simulink model "Pacemaker_Deliverable_1_Final_2023a"  (R2023a)
settings: Solver=FixedStepAuto  StartTime=0.0  StopTime=10.0  FixedStep=1e-3  RelTol=1e-3  EnableMultiTasking=on
undefined symbols (not defined in the file): D0, D1, D10, D11, D12, D13, D2, D3, D5, D6, D8, D9, PTA0, PTA1, PTA2, PTB9, PTC16, PTC17, PTC2, PTC4, PTD0, PTD1, PTD2, PTD3
libraries: frdmk64flib x14
settings Model: ExtModeTrigDuration=5  Creator=kelby  LastModifiedBy=kelby
settings OptimizationCC: EnhancedBackFolding=on  PassReuseOutputArgsAs=Individual arguments  ZeroExternalMemoryAtStartup=off  ZeroInternalMemoryAtStartup=off  MaxStackSize=64  OptimizeBlockOrder=speed  DifferentSizesBufferReuse=on  OptimizationCustomize=off  EfficientTunableParamExpr=on
settings DebuggingCC: ParameterTunabilityLossMsg=error
settings HardwareCC: ProdBitPerPointer=32  ProdBitPerSizeT=32  ProdBitPerPtrDiffT=32  ProdLargestAtomicInteger=Long  ProdLargestAtomicFloat=Double  ProdWordSize=32  ProdHWDeviceType=ARM Compatible->ARM Cortex
settings SFSimCC: MATLABDynamicMemAlloc=off
settings RTWCC: Description=Embedded Coder  SystemTargetFile=ert.tlc  HardwareBoard=NXP FRDM-K64F  TLCOptions="-aInlineSetEventsForThisBaseRateFcn=TLC_FALSE -aSuppressMultiTaskScheduler=TLC_FALSE  -aRateBasedStepFcn=0"  TemplateMakefile=ert_default_tmf  Toolchain=GNU Tools for ARM Embedded Processors
settings CodeAppCC: ForceParamTrailComments=on  IgnoreCustomStorageClasses=off  OperatorAnnotations=on  SimulinkDataObjDesc=on  SFDataObjDesc=on  InsertBlockDesc=on
settings ERTTargetCC: ExtModeTransport=4  ExtModeMexFile=sendToCommService

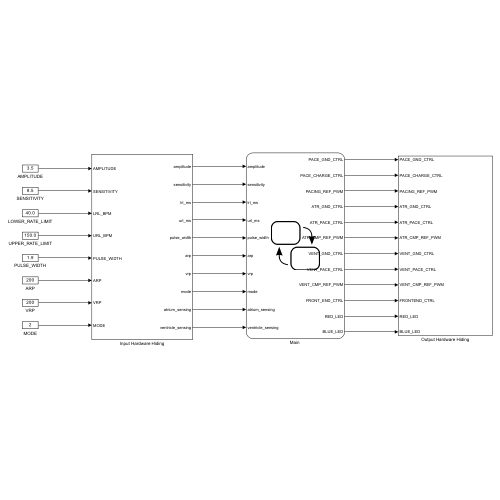
[thumbnail: Simulink's stored preview of the top-level diagram]
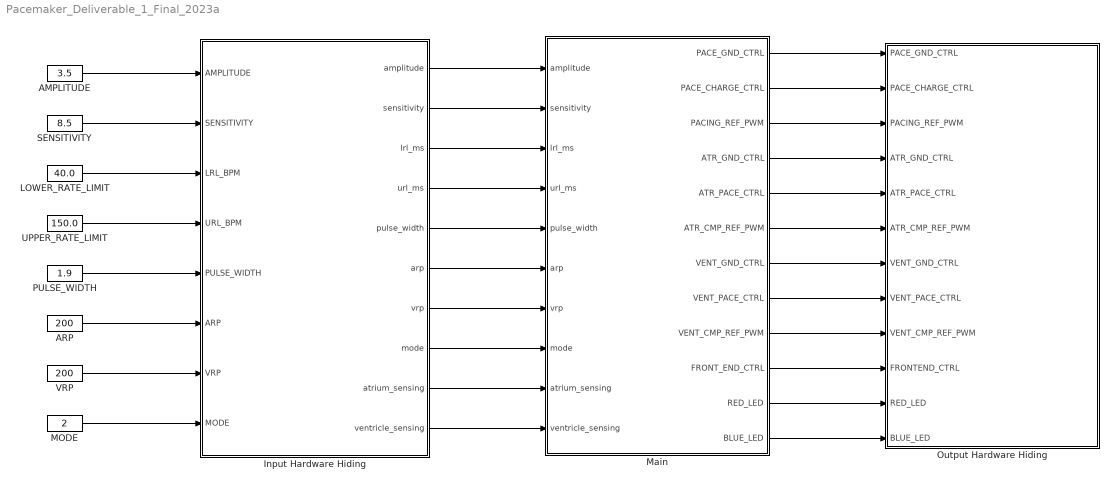
== system Pacemaker_Deliverable_1_Final_2023a ==
  AMPLITUDE : Constant  Value=3.5
  ARP : Constant  Value=200
  Input Hardware Hiding : Subsystem
  LOWER_RATE_LIMIT : Constant  Value=40.0
  MODE : Constant  Value=2
  "Main " : Stateflow chart  TreatAsAtomicUnit=on
  Output Hardware Hiding : Subsystem
  PULSE_WIDTH : Constant  Value=1.9
  SENSITIVITY : Constant  Value=8.5
  UPPER_RATE_LIMIT : Constant  Value=150.0
  VRP : Constant  Value=200
  wires:
  Input Hardware Hiding/1(amplitude) -> "Main "/1(amplitude)
  Input Hardware Hiding/3(lrl_ms) -> "Main "/3(lrl_ms)
  Input Hardware Hiding/4(url_ms) -> "Main "/4(url_ms)
  Input Hardware Hiding/5(pulse_width) -> "Main "/5(pulse_width)
  Input Hardware Hiding/8(mode) -> "Main "/8(mode)
  Input Hardware Hiding/6(arp) -> "Main "/6(arp)
  Input Hardware Hiding/7(vrp) -> "Main "/7(vrp)
  Input Hardware Hiding/2(sensitivity) -> "Main "/2(sensitivity)
  "Main "/4(ATR_GND_CTRL) -> Output Hardware Hiding/4(ATR_GND_CTRL)
  "Main "/5(ATR_PACE_CTRL) -> Output Hardware Hiding/5(ATR_PACE_CTRL)
  "Main "/2(PACE_CHARGE_CTRL) -> Output Hardware Hiding/2(PACE_CHARGE_CTRL)
  "Main "/1(PACE_GND_CTRL) -> Output Hardware Hiding/1(PACE_GND_CTRL)
  "Main "/3(PACING_REF_PWM) -> Output Hardware Hiding/3(PACING_REF_PWM)
  "Main "/7(VENT_GND_CTRL) -> Output Hardware Hiding/7(VENT_GND_CTRL)
  "Main "/8(VENT_PACE_CTRL) -> Output Hardware Hiding/8(VENT_PACE_CTRL)
  "Main "/9(VENT_CMP_REF_PWM) -> Output Hardware Hiding/9(VENT_CMP_REF_PWM)
  "Main "/6(ATR_CMP_REF_PWM) -> Output Hardware Hiding/6(ATR_CMP_REF_PWM)
  "Main "/12(BLUE_LED) -> Output Hardware Hiding/12(BLUE_LED)
  "Main "/11(RED_LED) -> Output Hardware Hiding/11(RED_LED)
  AMPLITUDE/1 -> Input Hardware Hiding/1(AMPLITUDE)
  LOWER_RATE_LIMIT/1 -> Input Hardware Hiding/3(LRL_BPM)
  UPPER_RATE_LIMIT/1 -> Input Hardware Hiding/4(URL_BPM)
  PULSE_WIDTH/1 -> Input Hardware Hiding/5(PULSE_WIDTH)
  MODE/1 -> Input Hardware Hiding/8(MODE)
  ARP/1 -> Input Hardware Hiding/6(ARP)
  VRP/1 -> Input Hardware Hiding/7(VRP)
  SENSITIVITY/1 -> Input Hardware Hiding/2(SENSITIVITY)
  Input Hardware Hiding/9(atrium_sensing) -> "Main "/9(atrium_sensing)
  Input Hardware Hiding/10(ventricle_sensing) -> "Main "/10(ventricle_sensing)
  "Main "/10(FRONT_END_CTRL) -> Output Hardware Hiding/10(FRONTEND_CTRL)

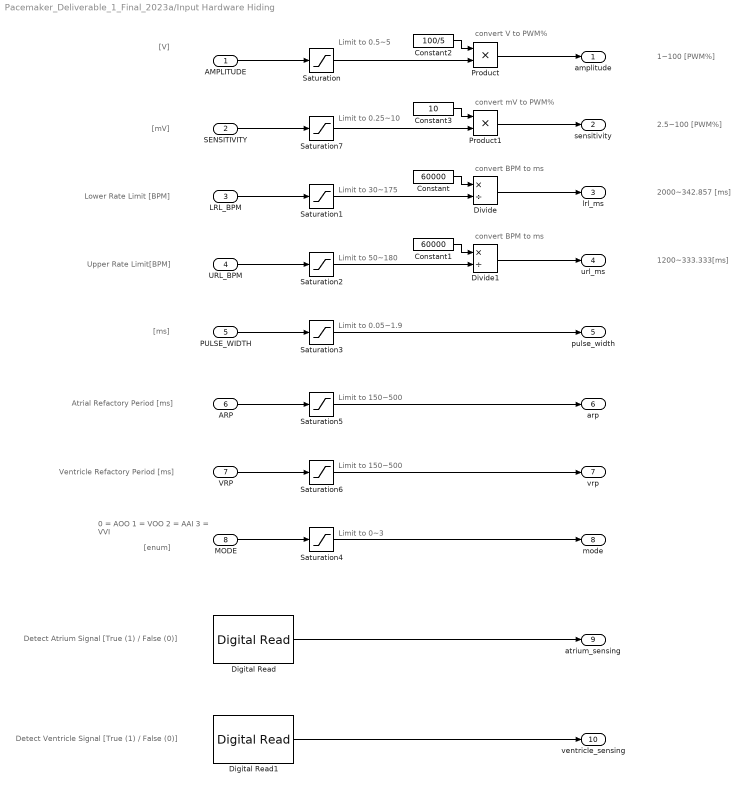
== system Pacemaker_Deliverable_1_Final_2023a/Input Hardware Hiding ==
  note: 0 = AOO
      | 1 = VOO
      | 2 = AAI
      | 3 = VVI
  note: Detect Atrium Signal [True (1) / False (0)]
  note: Limit to 0.5~5
  note: convert BPM to ms
  note: Ventricle Refactory Period [ms]
  note: Atrial Refactory Period [ms]
  note: convert BPM to ms
  note: Limit to 30~175
  note: Limit to 50~180
  note: Limit to 0.05~1.9
  note: Limit to 0~3
  note: Limit to 150~500
  note: Limit to 150~500
  note: Limit to 0.25~10
  note: convert V to PWM%
  note: convert mV to PWM%
  note: [mV]
  note: 2.5~100 [PWM%]
  note: 1~100 [PWM%]
  note: Lower Rate Limit [BPM]
  note: Upper Rate Limit[BPM]
  note: 2000~342.857 [ms]
  note: 1200~333.333[ms]
  note: [ms]
  note: [enum]
  note: [V]
  note: Detect Ventricle Signal [True (1) / False (0)]
  AMPLITUDE : Inport
  SENSITIVITY : Inport  Port=2
  LRL_BPM : Inport  Port=3
  URL_BPM : Inport  Port=4
  PULSE_WIDTH : Inport  Port=5
  ARP : Inport  Port=6
  VRP : Inport  Port=7
  MODE : Inport  Port=8
  Constant : Constant  Value=60000
  Constant1 : Constant  Value=60000
  Constant2 : Constant  Value=100/5
  Constant3 : Constant  Value=10
  Digital Read : frdmk64flib/Digital Read  Whichpin=PTC16 (D0)  SampleTime=-1
  Digital Read1 : frdmk64flib/Digital Read  Whichpin=PTC17 (D1)  SampleTime=-1
  Divide : Product  Inputs=*/
  Divide1 : Product  Inputs=*/
  Product : Product
  Product1 : Product
  Saturation : Saturate  UpperLimit=5  LowerLimit=0.5
  Saturation1 : Saturate  UpperLimit=175  LowerLimit=30
  Saturation2 : Saturate  UpperLimit=180  LowerLimit=50
  Saturation3 : Saturate  UpperLimit=1.9  LowerLimit=0.05
  Saturation4 : Saturate  UpperLimit=3  LowerLimit=0
  Saturation5 : Saturate  UpperLimit=500  LowerLimit=150
  Saturation6 : Saturate  UpperLimit=500  LowerLimit=150
  Saturation7 : Saturate  UpperLimit=10  LowerLimit=0.25
  amplitude : Outport
  sensitivity : Outport  Port=2
  lrl_ms : Outport  Port=3
  url_ms : Outport  Port=4
  pulse_width : Outport  Port=5
  arp : Outport  Port=6
  vrp : Outport  Port=7
  mode : Outport  Port=8
  atrium_sensing : Outport  Port=9
  ventricle_sensing : Outport  Port=10
  wires:
  AMPLITUDE/1 -> Saturation/1
  LRL_BPM/1 -> Saturation1/1
  Saturation1/1 -> Divide/2
  Constant/1 -> Divide/1
  Divide/1 -> lrl_ms/1
  URL_BPM/1 -> Saturation2/1
  PULSE_WIDTH/1 -> Saturation3/1
  Saturation3/1 -> pulse_width/1
  MODE/1 -> Saturation4/1
  Saturation4/1 -> mode/1
  ARP/1 -> Saturation5/1
  Saturation5/1 -> arp/1
  Saturation6/1 -> vrp/1
  VRP/1 -> Saturation6/1
  SENSITIVITY/1 -> Saturation7/1
  Digital Read1/1 -> ventricle_sensing/1
  Digital Read/1 -> atrium_sensing/1
  Constant1/1 -> Divide1/1
  Saturation2/1 -> Divide1/2
  Divide1/1 -> url_ms/1
  Saturation/1 -> Product/2
  Constant2/1 -> Product/1
  Product/1 -> amplitude/1
  Product1/1 -> sensitivity/1
  Saturation7/1 -> Product1/2
  Constant3/1 -> Product1/1

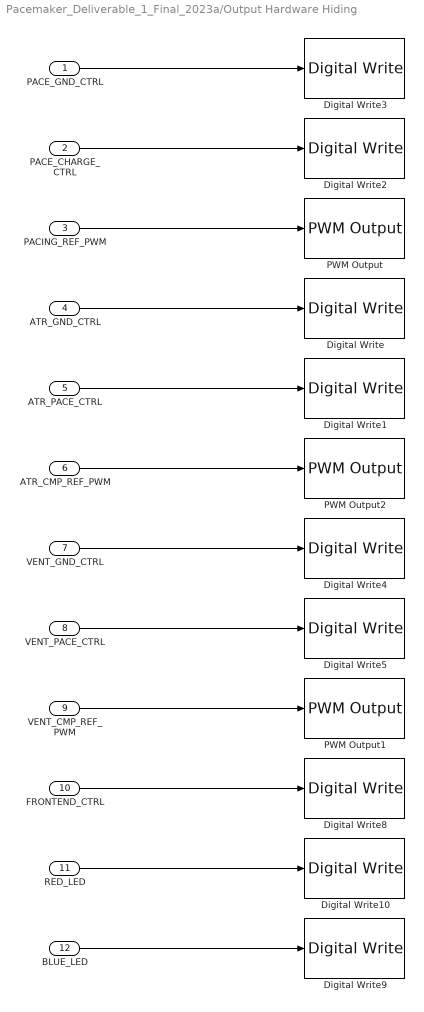
== system Pacemaker_Deliverable_1_Final_2023a/Output Hardware Hiding ==
  PACE_GND_CTRL : Inport
  PACE_CHARGE_CTRL : Inport  Port=2
  PACING_REF_PWM : Inport  Port=3
  ATR_GND_CTRL : Inport  Port=4
  ATR_PACE_CTRL : Inport  Port=5
  ATR_CMP_REF_PWM : Inport  Port=6
  VENT_GND_CTRL : Inport  Port=7
  VENT_PACE_CTRL : Inport  Port=8
  VENT_CMP_REF_PWM : Inport  Port=9
  FRONTEND_CTRL : Inport  Port=10
  RED_LED : Inport  Port=11
  BLUE_LED : Inport  Port=12
  Digital Write : frdmk64flib/Digital Write  Whichpin=PTD2 (D11)
  Digital Write1 : frdmk64flib/Digital Write  Whichpin=PTA0 (D8)
  Digital Write10 : frdmk64flib/Digital Write  Whichpin=RED_LED
  Digital Write2 : frdmk64flib/Digital Write  Whichpin=PTB9 (D2)
  Digital Write3 : frdmk64flib/Digital Write  Whichpin=PTD0 (D10)
  Digital Write4 : frdmk64flib/Digital Write  Whichpin=PTD3 (D12)
  Digital Write5 : frdmk64flib/Digital Write  Whichpin=PTC4 (D9)
  Digital Write8 : frdmk64flib/Digital Write  Whichpin=PTD1 (D13)
  Digital Write9 : frdmk64flib/Digital Write  Whichpin=BLUE_LED
  PWM Output : frdmk64flib/PWM Output  Whichpin=PTA2 (D5)  InitialFrequency=2000  InitialDutyCycle=0
  PWM Output1 : frdmk64flib/PWM Output  Whichpin=PTA1 (D3)  InitialFrequency=2000  InitialDutyCycle=0
  PWM Output2 : frdmk64flib/PWM Output  Whichpin=PTC2 (D6)  InitialFrequency=2000  InitialDutyCycle=0
  wires:
  VENT_GND_CTRL/1 -> Digital Write4/1
  PACE_GND_CTRL/1 -> Digital Write3/1
  VENT_PACE_CTRL/1 -> Digital Write5/1
  PACING_REF_PWM/1 -> PWM Output/1
  PACE_CHARGE_CTRL/1 -> Digital Write2/1
  ATR_PACE_CTRL/1 -> Digital Write1/1
  ATR_GND_CTRL/1 -> Digital Write/1
  VENT_CMP_REF_PWM/1 -> PWM Output1/1
  ATR_CMP_REF_PWM/1 -> PWM Output2/1
  BLUE_LED/1 -> Digital Write9/1
  RED_LED/1 -> Digital Write10/1
  FRONTEND_CTRL/1 -> Digital Write8/1

== stateflow chart Pacemaker_Deliverable_1_Final_2023a/Main  ==
  state AOO
    state AOO_Entry
      entry:
      % all ventricle controls set to 0
      PACING_REF_PWM = amplitude;
      PACE_GND_CTRL = 1;
      VENT_PACE_CTRL = 0;
      VENT_GND_CTRL = 0;
      RED_LED = 1;
      BLUE_LED = 0;
    state AOO_Pacing
      entry:
      % pacing atrium
      PACE_CHARGE_CTRL = 0;
      ATR_PACE_CTRL = 1;
      ATR_GND_CTRL = 0;
    state AOO_Charging
      entry:
      % charge C22, discharge C21
      PACE_CHARGE_CTRL = 1;
      ATR_PACE_CTRL = 0;
      ATR_GND_CTRL = 1;
    note: % total elapse time/cycle = lrl_ms
    (default) -> AOO_Entry
    AOO_Entry -> AOO_Charging
    AOO_Charging -> AOO_Pacing : [after(lrl_ms - pulse_width, msec)]
    AOO_Pacing -> AOO_Charging : [after(pulse_width, msec)]
  state VVI
    state VVI_Entry
      entry:
      % all atrium controls set to 0
      % ventricle variables set to be same as charging state to be ready for pacing
      PACING_REF_PWM = amplitude;
      VENT_CMP_REF_PWM = sensitivity;
      PACE_CHARGE_CTRL = 1;
      PACE_GND_CTRL = 1;
      ATR_PACE_CTRL = 0;
      ATR_GND_CTRL = 0;
      VENT_PACE_CTRL = 0;
      VENT_GND_CTRL = 1;
      BLUE_LED = 0;
      RED_LED = 0;
      heartbeat_detected = 0;
    state AAI_Charging
      entry:
      % charge C22, discharge C21
      PACE_CHARGE_CTRL = 1;
      VENT_PACE_CTRL = 0;
      VENT_GND_CTRL = 1;
    state VVI_Idle
      entry:
      % waiting for heartbeat / time to pace
      BLUE_LED = 0;
    state VVI_Detected
      entry:
      % heartbeat (ventricle) detected
      heartbeat_detected = 1;
    note: % total elapse time/cycle = lrl_ms
        | (regardless of heartbeat detected or not)
    state AAI_Pacing
      entry:
      % pacing ventricle
      PACE_CHARGE_CTRL = 0;
      VENT_PACE_CTRL = 1;
      VENT_GND_CTRL = 0;
      BLUE_LED = 1;
      heartbeat_detected = 0;
    (default) -> VVI_Entry
    VVI_Entry -> VVI_Idle
    VVI_Idle -> VVI_Detected [order 1] : [ventricle_sensing == 1]
    VVI.AAI_Charging -> VVI_Idle
    VVI_Detected -> VVI_Idle : [after(vrp, msec)]
    VVI_Idle -> VVI.AAI_Pacing [order 2] : [after(lrl_ms - pulse_width - heartbeat_detected * vrp, msec)]
    VVI.AAI_Pacing -> VVI.AAI_Charging : [after(pulse_width, msec)]
  state VOO
    state VOO_Entry
      entry:
      % all atrium controls set to 0
      PACING_REF_PWM = amplitude;
      PACE_GND_CTRL = 1;
      ATR_PACE_CTRL = 0;
      ATR_GND_CTRL = 0;
      RED_LED = 0;
      BLUE_LED = 1;
    state VOO_Charging
      entry:
      % charge C22, discharge C21
      PACE_CHARGE_CTRL = 1;
      VENT_PACE_CTRL = 0;
      VENT_GND_CTRL = 1;
    state VOO_Pacing
      entry:
      % pacing ventricle
      PACE_CHARGE_CTRL = 0;
      VENT_PACE_CTRL = 1;
      VENT_GND_CTRL = 0;
    note: % total elapse time/cycle = lrl_ms
    (default) -> VOO_Entry
    VOO_Entry -> VOO_Charging
    VOO_Charging -> VOO_Pacing : [after(lrl_ms - pulse_width, msec)]
    VOO_Pacing -> VOO_Charging : [after(pulse_width, msec)]
  state Idle
    entry:
    FRONT_END_CTRL = 1;
  state AAI
    state AAI_Entry
      entry:
      % all ventricle controls set to 0
      % atrium variables set to be same as charging state to be ready for pacing
      PACING_REF_PWM = amplitude;
      ATR_CMP_REF_PWM = sensitivity;
      PACE_CHARGE_CTRL = 1;
      PACE_GND_CTRL = 1;
      ATR_PACE_CTRL = 0;
      ATR_GND_CTRL = 1;
      VENT_PACE_CTRL = 0;
      VENT_GND_CTRL = 0;
      BLUE_LED = 0;
      RED_LED = 0;
      heartbeat_detected = 0;
    state AAI_Charging
      entry:
      % charge C22, discharge C21
      PACE_CHARGE_CTRL = 1;
      ATR_PACE_CTRL = 0;
      ATR_GND_CTRL = 1;
    state AAI_Idle
      entry:
      % waiting for heartbeat / time to pace
      RED_LED = 0;
    state AAI_Detected
      entry:
      % heartbeat (atrium) detected
      heartbeat_detected = 1;
    note: % total elapse time/cycle = lrl_ms
        | (regardless of heartbeat detected or not)
    state AAI_Pacing
      entry:
      % pacing atrium
      PACE_CHARGE_CTRL = 0;
      ATR_PACE_CTRL = 1;
      ATR_GND_CTRL = 0;
      RED_LED = 1;
      heartbeat_detected = 0;
    (default) -> AAI_Entry
    AAI_Entry -> AAI_Idle
    AAI_Idle -> AAI_Detected [order 1] : [atrium_sensing == 1]
    AAI.AAI_Charging -> AAI_Idle
    AAI_Detected -> AAI_Idle : [after(arp, msec)]
    AAI_Idle -> AAI.AAI_Pacing [order 2] : [after(lrl_ms - pulse_width - heartbeat_detected * arp, msec)]
    AAI.AAI_Pacing -> AAI.AAI_Charging : [after(pulse_width, msec)]
  AOO -> Idle : [mode ~= 0]
  Idle -> AOO [order 1] : [mode == 0]
  (default) -> Idle
  VOO -> Idle : [mode ~= 1]
  Idle -> VVI [order 4] : [mode == 3]
  Idle -> VOO [order 2] : [mode == 1]
  VVI -> Idle : [mode ~= 3]
  Idle -> AAI [order 3] : [mode == 2]
  AAI -> Idle : [mode ~= 2]
  data: PACE_GND_CTRL output; PACE_CHARGE_CTRL output; PACING_REF_PWM output; amplitude input; sensitivity input; lrl_ms input; url_ms input; pulse_width input; arp input; vrp input; mode input; atrium_sensing input; ventricle_sensing input; ATR_GND_CTRL output; ATR_PACE_CTRL output; ATR_CMP_REF_PWM output; VENT_GND_CTRL output; VENT_PACE_CTRL output; VENT_CMP_REF_PWM output; FRONT_END_CTRL output; RED_LED output; BLUE_LED output; heartbeat_detected local
